simulink model "untitled"  (R2013a)
settings: Solver=ode45  StartTime=0.0  StopTime=10.0  RelTol=1e-3
values from neighbouring files (symbols this model uses):
  A = [-1.064 1.000; 290.26 0.00]    [GNC.m]
  B = [-0.25; -331.40]    [GNC.m]
  C = [-123.34 0.00; 0.00 1.00]    [GNC.m]
  D = [-13.51; 0]    [GNC.m]
  dT1 = 0.75    [GNC.m]
  dT2 = 0.25    [GNC.m]
  ELEV_INIT = 10000    [GNC.m]
  ELEV_TARGET = 795    [GNC.m]
  LAT_INIT = 34.2329    [GNC.m]
  LAT_OBS = 34.61916    [GNC.m]
  LAT_TARGET = 34.6588    [GNC.m]
  LON_INIT = -119.4573    [GNC.m]
  LON_OBS = -118.8429    [GNC.m]
  LON_TARGET = -118.79745    [GNC.m]
  vel = 1021.08    [GNC.m]
undefined symbols (not defined in the file or in its folder): Earth, K, L, WGS84
libraries: simulink x4, aerolibtransform2 x1
settings Model: Creator=SAI  LastModifiedBy=SAI
settings DataIOCC: InspectSignalLogs=on

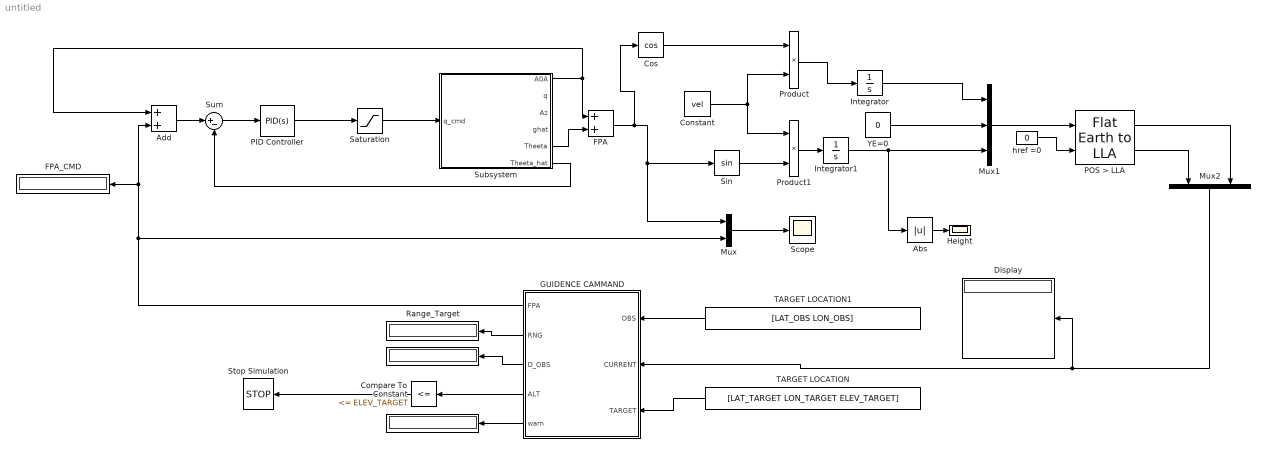
== system untitled ==
  " " : Display
  " " : Display
  " Range_Target " : Display
  Abs : Abs
  Add : Sum
  Compare To Constant : simulink/Logic and Bit Operations/Compare To Constant  relop=<=  const=ELEV_TARGET  OutDataTypeStr=boolean
  Constant : Constant  Value=vel
  Cos : Trigonometry  Operator=cos
  Display : Display
  FPA : Sum
  FPA_CMD : Display
  GUIDENCE CAMMAND : MATLAB Function  TreatAsAtomicUnit=on
  Height : Scope
      settings: SaveName=ScopeData2
  Integrator : Integrator
  Integrator1 : Integrator  InitialCondition=-ELEV_INIT
  Mux : Mux  Inputs=2
  Mux1 : Mux  Inputs=3
  Mux2 : Mux  Inputs=2
  PID Controller : simulink/Continuous/PID Controller  Controller=PID  TimeDomain=Continuous-time  SampleTime=1  IntegratorMethod=Forward Euler  FilterMethod=Forward Euler  Form=Parallel  P=-1  I=0  D=0  N=100  InitialConditionSource=internal  InitialConditionForIntegrator=0  InitialConditionForFilter=0  ExternalReset=none  LimitOutput=off  UpperSaturationLimit=inf  LowerSaturationLimit=-inf  LinearizeAsGain=on  AntiWindupMode=none  Kb=1  TrackingMode=off  Kt=1  PParamMin=[]  PParamMax=[]  IParamMin=[]  IParamMax=[]  DParamMin=[]  DParamMax=[]  NParamMin=[]  NParamMax=[]  KbParamMin=[]  KbParamMax=[]  KtParamMin=[]  KtParamMax=[]  POutMin=[]  POutMax=[]  IOutMin=[]  IOutMax=[]  DOutMin=[]  DOutMax=[]  NOutMin=[]  NOutMax=[]  KbOutMin=[]  KbOutMax=[]  KtOutMin=[]  KtOutMax=[]  IntegratorOutMin=[]  IntegratorOutMax=[]  FilterOutMin=[]  FilterOutMax=[]  SumOutMin=[]  SumOutMax=[]  SumI1OutMin=[]  SumI1OutMax=[]  SumI2OutMin=[]  SumI2OutMax=[]  SumI3OutMin=[]  SumI3OutMax=[]  SumDOutMin=[]  SumDOutMax=[]  SaturationOutMin=[]  SaturationOutMax=[]  IntegratorContinuousStateAttributes=''  IntegratorStateMustResolveToSignalObject=off  IntegratorRTWStateStorageClass=Auto  FilterContinuousStateAttributes=''  FilterStateMustResolveToSignalObject=off  FilterRTWStateStorageClass=Auto
  POS > LLA : aerolibtransform2/Flat Earth to LLA  units=Metric (MKS)  ptype=Earth (WGS84)  F=1/298.257223563  R=6378137  LL0=[LAT_INIT LON_INIT]  psi=yaw_init
  Product : Product
  Product1 : Product
  Saturation : Saturate
  Scope : Scope
  Sin : Trigonometry
  Stop Simulation : Stop
  Subsystem : Subsystem
  Sum : Sum  Inputs=|+-
  TARGET LOCATION : Constant  Value=[LAT_TARGET LON_TARGET ELEV_TARGET]
  TARGET LOCATION1 : Constant  Value=[LAT_OBS LON_OBS]
  "YE=0 " : Constant  Value=0
  href =0 : Constant  Value=0
  wires:
  Saturation/1 -> Subsystem/1("q_cmd ")
  PID Controller/1 -> Saturation/1
  Sum/1 -> PID Controller/1
  Subsystem/6("Theeta_hat ") -> Sum/2
  Add/1 -> Sum/1
  Subsystem/1("A0A ") -> Add/1, FPA/1
  Subsystem/5(Theeta) -> FPA/2
  FPA/1 -> Cos/1, Sin/1, Mux/1
  Mux/1 -> Scope/1
  Cos/1 -> Product/1
  Constant/1 -> Product1/1, Product/2
  Product/1 -> Integrator/1
  Product1/1 -> Integrator1/1
  Integrator/1 -> Mux1/1
  "YE=0 "/1 -> Mux1/2
  Integrator1/1 -> Abs/1, Mux1/3
  Abs/1 -> Height/1
  Mux1/1 -> POS > LLA/1
  href =0/1 -> POS > LLA/2
  POS > LLA/2 -> Mux2/1
  POS > LLA/1 -> Mux2/2
  TARGET LOCATION/1 -> GUIDENCE CAMMAND/3(TARGET)
  Mux2/1 -> Display/1, GUIDENCE CAMMAND/2(CURRENT)
  GUIDENCE CAMMAND/5(warn) -> " "/1
  GUIDENCE CAMMAND/3(D_OBS) -> " "/1
  GUIDENCE CAMMAND/2(RNG) -> " Range_Target "/1
  GUIDENCE CAMMAND/1(FPA) -> FPA_CMD/1, Add/2, Mux/2
  GUIDENCE CAMMAND/4(ALT) -> Compare To Constant/1
  Compare To Constant/1 -> Stop Simulation/1
  Sin/1 -> Product1/2
  TARGET LOCATION1/1 -> GUIDENCE CAMMAND/1(OBS)

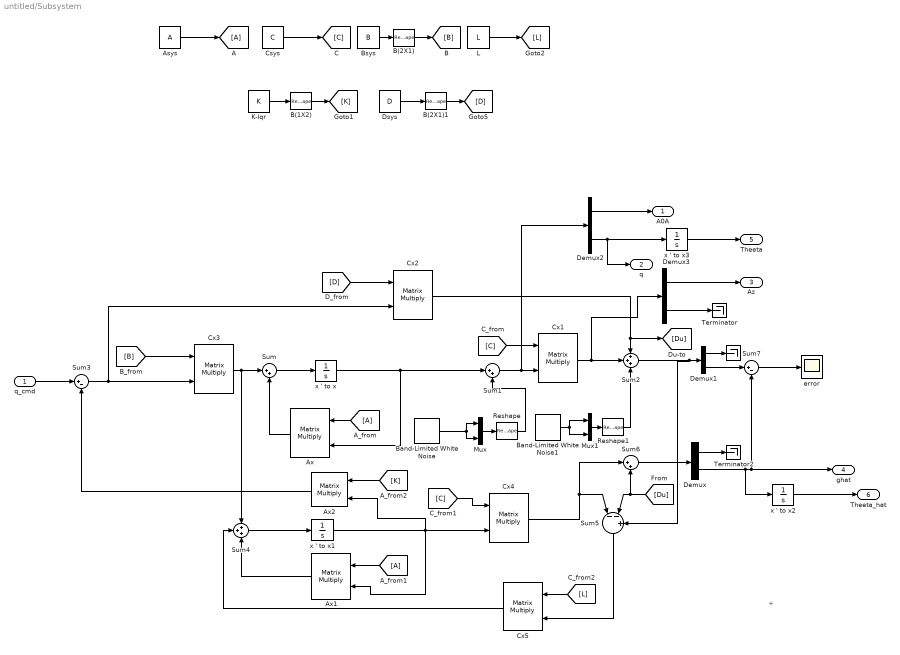
== system untitled/Subsystem ==
  note: +
  "q_cmd " : Inport
  " " : Terminator
  Asys : Constant  Value=A
  Ax : Product  Multiplication=Matrix(*)
  Ax1 : Product  Multiplication=Matrix(*)
  Ax2 : Product  Multiplication=Matrix(*)
  B(1X2) : Reshape  OutputDimensionality=Customize  OutputDimensions=[1,2]
  B(2X1) : Reshape  OutputDimensionality=Customize  OutputDimensions=[2,1]
  B(2X1)1 : Reshape  OutputDimensionality=Customize  OutputDimensions=[2,1]
  Band-Limited White Noise : simulink/Sources/Band-Limited White Noise  Cov=[0.00000001]  Ts=dT1  seed=[23341]
  Band-Limited White Noise1 : simulink/Sources/Band-Limited White Noise  Cov=[0.00001]  Ts=dT2  seed=[23341]
  Bsys : Constant  Value=B
  Csys : Constant  Value=C
  Cx{1..5} (5 alike) : Product  Multiplication=Matrix(*)
  Demux{,1..3} (4 alike) : Demux  Outputs=2
  Dsys : Constant  Value=D
  K-lqr : Constant  Value=K
  L : Constant  Value=L
  Mux : Mux  Inputs=2
  Mux1 : Mux  Inputs=2
  Reshape : Reshape  OutputDimensionality=Customize  OutputDimensions=[2,1]
  Reshape1 : Reshape  OutputDimensionality=Customize  OutputDimensions=[2,1]
  Sum : Sum  Inputs=|++
  Sum1 : Sum  Inputs=|++
  Sum2 : Sum  Inputs=+++
  Sum3 : Sum  Inputs=|+-
  Sum4 : Sum  Inputs=+++
  Sum5 : Sum  Inputs=|--+
  Sum6 : Sum  Inputs=|++
  Sum7 : Sum  Inputs=|+-
  Terminator : Terminator
  Terminator2 : Terminator
  error : Scope
  x ' to x{,1..3} (4 alike) : Integrator
  "A0A " : Outport
  q : Outport  Port=2
  "Az " : Outport  Port=3
  "ghat " : Outport  Port=4
  Theeta : Outport  Port=5
  "Theeta_hat " : Outport  Port=6
  wires:
  x ' to x3/1 -> Theeta/1
  [B] -> Cx3/1
  Sum1/1 -> Demux2/1, Cx1/2
  Bsys/1 -> B(2X1)/1
  [K] -> Ax2/1
  [C] -> Cx1/1
  Cx3/1 -> Sum/1, Sum4/1
  Ax/1 -> Sum/2
  [D] -> Cx2/1
  Sum/1 -> x ' to x/1
  x ' to x/1 -> Sum1/1, Ax/2
  Reshape/1 -> Sum1/2
  Sum4/1 -> x ' to x1/1
  Mux1/1 -> Reshape1/1
  Band-Limited White Noise/1 -> Mux/1, Mux/2
  Demux2/1 -> "A0A "/1
  K-lqr/1 -> B(1X2)/1
  Cx4/1 -> Sum5/1, Sum6/1
  Ax1/1 -> Sum4/3
  [Du] -> Sum6/2, Sum5/2
  B(1X2)/1 -> [K]
  Sum5/1 -> Cx5/2
  Band-Limited White Noise1/1 -> Mux1/1, Mux1/2
  Ax2/1 -> Sum3/2
  Demux3/2 -> Terminator/1
  Demux1/2 -> Sum7/1
  "q_cmd "/1 -> Sum3/1
  Mux/1 -> Reshape/1
  [A] -> Ax/1
  Asys/1 -> [A]
  Demux/2 -> "ghat "/1, Sum7/2, x ' to x2/1
  Demux2/2 -> q/1, x ' to x3/1
  Dsys/1 -> B(2X1)1/1
  [L] -> Cx5/1
  Reshape1/1 -> Sum2/3
  Sum7/1 -> error/1
  [C] -> Cx4/1
  Csys/1 -> [C]
  Sum2/1 -> Demux1/1, Sum5/3
  Sum3/1 -> Cx2/2, Cx3/2
  L/1 -> [L]
  Cx5/1 -> Sum4/2
  Demux1/1 -> " "/1
  Demux/1 -> Terminator2/1
  x ' to x2/1 -> "Theeta_hat "/1
  Cx1/1 -> Demux3/1, Sum2/2
  [A] -> Ax1/1
  B(2X1)/1 -> [B]
  Cx2/1 -> [Du], Sum2/1
  B(2X1)1/1 -> [D]
  Sum6/1 -> Demux/1
  Demux3/1 -> "Az "/1
  x ' to x1/1 -> Ax2/2, Cx4/2, Ax1/2

== matlab function untitled/GUIDENCE CAMMAND ==
  data: OBS input; FPA output; CURRENT input; TARGET input; RNG output; D_OBS output; ALT output; warn output
function [FPA,RNG,D_OBS,ALT,warn]= fcn(OBS,CURRENT,TARGET)
%#codegen
R=6.371e3;
d2r=pi/180;
LAT_OBS = OBS(1);
LON_OBS = OBS(2);
thres =2000;
LAT_TARGET = TARGET(1);
LON_TARGET = TARGET(2);
ELEV_TARGET = TARGET(3);

ELEV_CUR =CURRENT(1);
LAT_CUR=CURRENT(2);
LON_CUR=CURRENT(3);

l1=LAT_CUR*d2r;
u1=LON_CUR*d2r;
l2=LAT_TARGET*d2r;
u2=LON_TARGET*d2r;
dh=abs(ELEV_TARGET-ELEV_CUR);

dl=l2-l1;
du=u2-u1;
a=sin(dl/2)^2+cos(l1)*cos(l2)*sin(du/2)^2;
c=2*atan2(sqrt(a),sqrt(1-a));
d=R*c;
l3=LAT_OBS*d2r;
u3=LON_OBS*d2r;
a=sin(dl/2)^2+cos(l1)*cos(l2)*sin(du/2)^2;
c=2*atan2(sqrt(a),sqrt(1-a));
d_obs=R*c;
range=sqrt(d^2+dh^2);
if abs(d_obs)>=thres
    w=0;
    FPA_CMD =atan(dh/d);
else
    w=1;
    FPA_CMD=0;
end
    FPA=FPA_CMD;
    RNG = range;
    D_OBS = d_obs;
    warn =w;
    ALT =ELEV_CUR;
